simulink model "IMUdataFinalr3PDs0x2810x29"  (R2024a)
settings: Solver=FixedStepAuto  StartTime=0.0  StopTime=100  FixedStep=.01  RelTol=1e-3  EnableMultiTasking=on
libraries: instrumentlib x2, hdlsllib x1, instrumentseriallib x1
settings Model: Creator=juanandrespelaezb  LastModifiedBy=NYCST
settings SolverCC: PositivePriorityOrder=on  AutoInsertRateTranBlk=on
settings OptimizationCC: EnhancedBackFolding=on  PassReuseOutputArgsThreshold=0  MaxStackSize=64  OptimizeBlockOrder=speed  DifferentSizesBufferReuse=on  OptimizationCustomize=off
settings DebuggingCC: ParameterTunabilityLossMsg=error
settings HardwareCC: ProdBitPerLong=64  ProdLargestAtomicInteger=LongLong  ProdLargestAtomicFloat=Double  ProdLongLongMode=on  ProdHWDeviceType=ARM Compatible->ARM 64-bit (LP64)
settings RTWCC: Description=Embedded Coder  SystemTargetFile=ert.tlc  HardwareBoard=Raspberry Pi (64bit)  TLCOptions="-aInlineSetEventsForThisBaseRateFcn=TLC_FALSE -aSuppressMultiTaskScheduler=TLC_FALSE  -aRateBasedStepFcn=0"  TemplateMakefile=ert_default_tmf  Toolchain=GNU GCC Embedded Linux  BuildConfiguration=Faster Runs
settings CodeAppCC: ForceParamTrailComments=on  OperatorAnnotations=on
settings ERTTargetCC: ERTCustomFileBanners=off  SupportContinuousTime=on  SupportNonInlinedSFcns=on  RemoveResetFunc=off  SupportVariableSizeSignals=on  ModelStepFunctionPrototypeControlCompliant=off  ExtModeTransport=2  ExtModeStaticAlloc=on  ExtModeMexFile=ext_xcp  ExtModeIntrfLevel=Level2 - Open

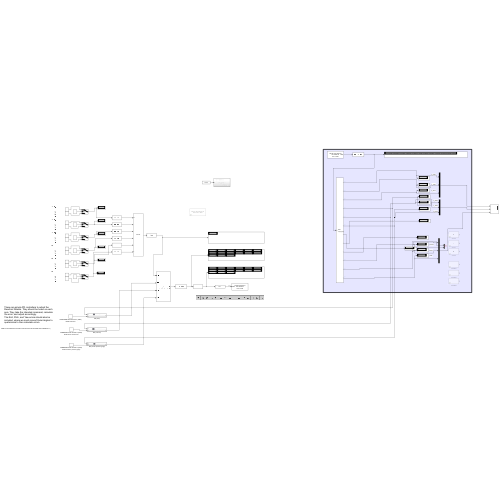
[thumbnail: Simulink's stored preview of the top-level diagram]
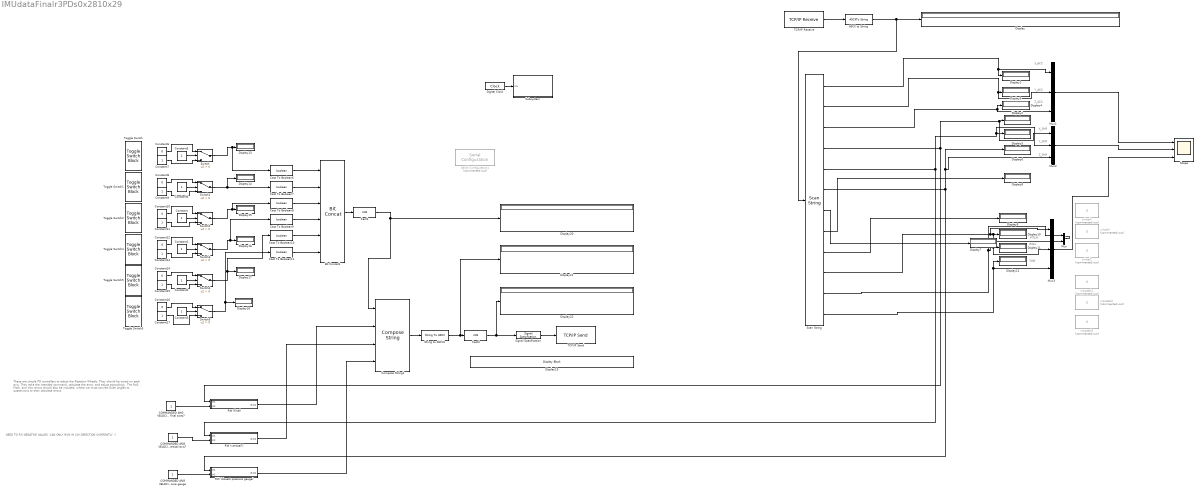
== system IMUdataFinalr3PDs0x2810x29 ==
  note: NEED TO FIX NEGATIVE VALUES. CAN ONLY RUN IN CW DIRECTION CURRENTLY :(
  note: These are simple PD controllers to adjust the Reaction Wheels. They should be tuned on each axis. They take the intended command, calculate the error, and adjust accordingly.
      | The Roll, Pitch, and Yaw errors should also be included, where we must convert Euler Angles to quaternions to then calculate errors.
  note: ROLL
  note: Z_GYR
  note: PITCH
  note: YAW
  note: Y_GYR
  note: X_GYR
  note: Z_ACC
  note: Y_ACC
  note: X_ACC
  ASCII to String : ASCIIToString
  Bit Concat1 : hdlsllib/Logic and Bit Operations/Bit Concat  numInputs=6
  COMMANDED ANG VELOCITY (PWM) IN RW about vertical axis? : Constant
  COMMANDED ANG VELOCITY (PWM) IN RW closest to pressure gauge : Constant
  COMMANDED ANG VELOCITY (PWM) IN RW final axes? : Constant
  Cast To Boolean{6..11} (6 alike) : DataTypeConversion  OutDataTypeStr=boolean  SaturateOnIntegerOverflow=off  RndMeth=Floor
  Cast1 : DataTypeConversion  OutDataTypeStr=int8  SaturateOnIntegerOverflow=off  RndMeth=Floor
  Cast4 : DataTypeConversion  OutDataTypeStr=int8  SaturateOnIntegerOverflow=off  RndMeth=Floor
  Compose String1 : ComposeString  Format="\"%02d;%03d;%03d;%03d\\n\""
  Constant{,1..5,7,9,11,13,15,17} (12 alike) : Constant
  Constant{6,8,10,12,14,16} (6 alike) : Constant  Value=0
  Digital Clock : DigitalClock
  Display{,1..18,20..22} (22 alike) : Display
  Display19 : DisplayBlock  LabelPosition=Hide  Format=long  Transparency=1
  Mux : Mux  Inputs=2
  Mux1 : Mux  Inputs=3
  Mux2 : Mux  Inputs=3
  Mux3 : Mux  Inputs=3
  RW (closest pressure gauge) : Subsystem
  RW (final) : Subsystem
  RW (vertical?) : Subsystem
  Scan String : ScanString  Format="\"%f,%f,%f,%f,%f,%f,%f,%f,%f,%f,%f,%f\""
  Scope : Scope  NumInputPorts=3
  Serial Configuration1 : instrumentseriallib/Serial Configuration  Priority=-200000  Commented=on  PortSel=/dev/cu.usbmodem2101  Port=/dev/cu.usbmodem2101  ComPort=/dev/cu.usbmodem2101  BaudRate=9600  DataBits=8  Parity=none  StopBits=1  ByteOrder=little-endian  FlowControl=none  Timeout=10  SimulateUsing=Interpreted execution  BlockInModel=on  aMode=1
  Signal Specification : SignalSpecification  SampleTime=.1
      settings: LockScale=on
  String to ASCII1 : StringToASCII  OutputVectorSize=15
  Subsystem : Subsystem
  Switch{,1..5} (6 alike) : Switch  Criteria=u2 > Threshold  SaturateOnIntegerOverflow=off  InputSameDT=off
  TCP/IP Receive : instrumentlib/TCP//IP Receive  Host=192.168.86.21  Port=12345  DataSize=[ 120, 1 ]  DataType=uint8  ASCIIFormatting=%f  Terminator=LF  CustomTerminator=10  ByteOrder=big-endian  EnableBlockingMode=on  Timeout=10  SampleTime=0.01  SimulateUsing=Interpreted execution
  TCP/IP Send : instrumentlib/TCP//IP Send  Host=192.168.86.21  Port=12345  ByteOrder=big-endian  EnableBlockingMode=on  Timeout=10  TransferDelay=on  SimulateUsing=Interpreted execution
  Toggle Switch{,1..5} (6 alike) : ToggleSwitchBlock
      settings: Values={{'Off', 'On'}, [0 1]}
  massBal1 : Constant  Commented=on  Value=0
  massBal2 : Constant  Commented=on  Value=0
  massBal3 : Constant  Commented=on  Value=0
  wheelX : Constant  Commented=on  Value=0
  wheelY : Constant  Commented=on  Value=0
  wheelZ : Constant  Commented=on  Value=0
  wires:
  Mux/1 -> ?
  Scan String/2 -> Mux1/2, Display3/1
  ASCII to String/1 -> Scan String/1, Display/1
  Scan String/7 -> Display7/1
  Scan String/1 -> Display1/1, Mux1/1
  Mux2/1 -> Scope/2
  Scan String/11 -> Mux/1, Mux3/2, Display11/1
  Mux1/1 -> Scope/1
  Scan String/6 -> Mux2/3, Display6/1, RW (closest pressure gauge)/1(In1)
  Scan String/3 -> Mux1/3, Display4/1
  Scan String/5 -> RW (vertical?)/1(In1), Mux2/2, Display5/1
  Scan String/8 -> Display8/1
  Scan String/4 -> RW (final)/1(In1), Display2/1, Mux2/1
  Scan String/9 -> Display9/1
  Scan String/12 -> Display12/1, Mux3/3
  Scan String/10 -> Mux3/1, Mux/2, Display10/1
  Digital Clock/1 -> Subsystem/1(In1)
  TCP/IP Receive/1 -> ASCII to String/1
  Constant6/1 -> Switch/1
  Constant7/1 -> Switch/3
  Constant8/1 -> Switch1/1
  Constant9/1 -> Switch1/3
  Constant10/1 -> Switch2/1
  Constant11/1 -> Switch2/3
  Constant13/1 -> Switch3/3
  Constant12/1 -> Switch3/1
  Constant14/1 -> Switch4/1
  Constant15/1 -> Switch4/3
  Constant16/1 -> Switch5/1
  Constant17/1 -> Switch5/3
  Constant/1 -> Switch2/2
  Constant1/1 -> Switch3/2
  Constant2/1 -> Switch4/2
  Constant3/1 -> Switch5/2
  Constant4/1 -> Switch1/2
  Constant5/1 -> Switch/2
  Switch/1 -> Cast To Boolean6/1, Display13/1
  Switch1/1 -> Cast To Boolean7/1, Display14/1
  Switch2/1 -> Cast To Boolean8/1, Display15/1
  Switch3/1 -> Cast To Boolean9/1, Display16/1
  Switch4/1 -> Cast To Boolean10/1, Display17/1
  Switch5/1 -> Cast To Boolean11/1, Display18/1
  Cast To Boolean9/1 -> Bit Concat1/4
  Cast To Boolean7/1 -> Bit Concat1/2
  Cast To Boolean10/1 -> Bit Concat1/5
  Cast To Boolean6/1 -> Bit Concat1/1
  Cast To Boolean8/1 -> Bit Concat1/3
  Cast To Boolean11/1 -> Bit Concat1/6
  Bit Concat1/1 -> Cast1/1
  Cast1/1 -> Compose String1/1, Display20/1
  Compose String1/1 -> String to ASCII1/1
  String to ASCII1/1 -> Display21/1, Cast4/1
  Cast4/1 -> Display22/1, Signal Specification/1
  Signal Specification/1 -> TCP/IP Send/1
  Mux3/1 -> Scope/3
  COMMANDED ANG VELOCITY (PWM) IN RW closest to pressure gauge/1 -> RW (closest pressure gauge)/2(In2)
  RW (closest pressure gauge)/1(Out1) -> Compose String1/4
  COMMANDED ANG VELOCITY (PWM) IN RW about vertical axis?/1 -> RW (vertical?)/2(In2)
  RW (vertical?)/1(Out1) -> Compose String1/3
  COMMANDED ANG VELOCITY (PWM) IN RW final axes?/1 -> RW (final)/2(In2)
  RW (final)/1(Out1) -> Compose String1/2

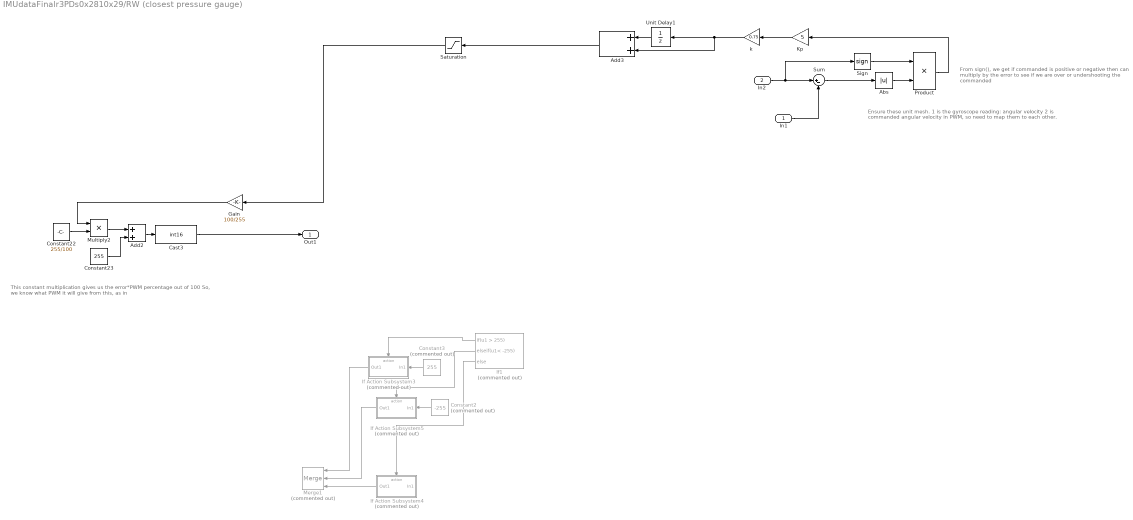
== system IMUdataFinalr3PDs0x2810x29/RW (closest pressure gauge) ==
  note: This constant multiplication gives us the error*PWM percentage out of 100
      | So, we know what PWM it will give from this, as in
  note: From sign(), we get if commanded is positive or negative
      | then can multiply by the error to see if we are over or undershooting
      | the commanded
  note: Ensure these unit mesh. 1 is the gyroscope reading: angular velocity
      | 2 is commanded angular velocity in PWM, so need to map them to each other.
  In1 : Inport
  In2 : Inport  Port=2
  Abs : Abs  SaturateOnIntegerOverflow=off
  Add2 : Sum
  Add3 : Sum
  Cast3 : DataTypeConversion  OutDataTypeStr=int16  SaturateOnIntegerOverflow=off  RndMeth=Floor
  Constant2 : Constant  Commented=on  Value=-255
  Constant22 : Constant  Value=255/100
  Constant23 : Constant  Value=255
  Constant3 : Constant  Commented=on  Value=255
  Gain : Gain  Gain=100/255
  If Action Subsystem3 : Subsystem  Commented=on  TreatAsAtomicUnit=on
  If Action Subsystem4 : Subsystem  Commented=on  TreatAsAtomicUnit=on
  If Action Subsystem5 : Subsystem  Commented=on  TreatAsAtomicUnit=on
  If1 : If  Commented=on  IfExpression=u1 > 255  ElseIfExpressions=u1< -255
  Kp : Gain  Gain=5
  Merge1 : Merge  Commented=on  Inputs=3
  Multiply2 : Product
  Product : Product
  Saturation : Saturate  UpperLimit=255  LowerLimit=-255
  Sign : Signum
  Sum : Sum  Inputs=|+-
  Unit Delay1 : UnitDelay  SampleTime=-1  HasFrameUpgradeWarning=on
  k : Gain  Gain=0.75
  Out1 : Outport
  wires:
  Multiply2/1 -> Add2/1
  Gain/1 -> Multiply2/1
  Constant23/1 -> Add2/2
  k/1 -> Add3/2, Unit Delay1/1
  Sum/1 -> Abs/1
  Unit Delay1/1 -> Add3/1
  Add2/1 -> Cast3/1
  Constant22/1 -> Multiply2/2
  Saturation/1 -> Gain/1
  Kp/1 -> k/1
  In1/1 -> Sum/2
  Cast3/1 -> Out1/1
  In2/1 -> Sign/1, Sum/1
  Sign/1 -> Product/1
  Abs/1 -> Product/2
  Product/1 -> Kp/1
  If1/2 -> If Action Subsystem5/Action
  Constant2/1 -> If Action Subsystem5/1(In1)
  Constant3/1 -> If Action Subsystem3/1(In1)
  If1/1 -> If Action Subsystem3/Action
  If Action Subsystem5/1(Out1) -> Merge1/2
  ? -> If Action Subsystem4/1(In1), If1/1
  If Action Subsystem3/1(Out1) -> Merge1/1
  If1/3 -> If Action Subsystem4/Action
  If Action Subsystem4/1(Out1) -> Merge1/3
  Add3/1 -> Saturation/1

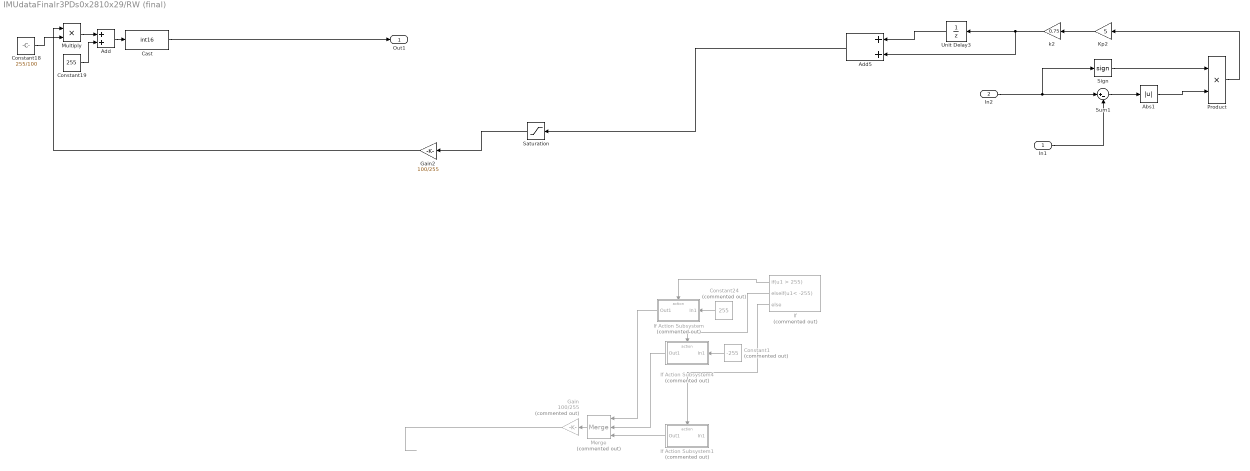
== system IMUdataFinalr3PDs0x2810x29/RW (final) ==
  In1 : Inport
  In2 : Inport  Port=2
  Abs1 : Abs  SaturateOnIntegerOverflow=off
  Add : Sum
  Add5 : Sum
  Cast : DataTypeConversion  OutDataTypeStr=int16  SaturateOnIntegerOverflow=off  RndMeth=Floor
  Constant1 : Constant  Commented=on  Value=-255
  Constant18 : Constant  Value=255/100
  Constant19 : Constant  Value=255
  Constant24 : Constant  Commented=on  Value=255
  Gain : Gain  Commented=on  Gain=100/255
  Gain2 : Gain  Gain=100/255
  If : If  Commented=on  IfExpression=u1 > 255  ElseIfExpressions=u1< -255
  If Action Subsystem : Subsystem  Commented=on  TreatAsAtomicUnit=on
  If Action Subsystem1 : Subsystem  Commented=on  TreatAsAtomicUnit=on
  If Action Subsystem4 : Subsystem  Commented=on  TreatAsAtomicUnit=on
  Kp2 : Gain  Gain=5
  Merge : Merge  Commented=on  Inputs=3
  Multiply : Product
  Product : Product
  Saturation : Saturate  UpperLimit=255  LowerLimit=-255
  Sign : Signum
  Sum1 : Sum  Inputs=|+-
  Unit Delay3 : UnitDelay  SampleTime=-1  HasFrameUpgradeWarning=on
  k2 : Gain  Gain=0.75
  Out1 : Outport
  wires:
  Constant19/1 -> Add/2
  Constant18/1 -> Multiply/2
  Unit Delay3/1 -> Add5/1
  Multiply/1 -> Add/1
  Saturation/1 -> Gain2/1
  Add/1 -> Cast/1
  In2/1 -> Sign/1, Sum1/1
  Kp2/1 -> k2/1
  Cast/1 -> Out1/1
  k2/1 -> Add5/2, Unit Delay3/1
  Sum1/1 -> Abs1/1
  In1/1 -> Sum1/2
  Gain2/1 -> Multiply/1
  Gain/1 -> ?
  If/3 -> If Action Subsystem1/Action
  If Action Subsystem/1(Out1) -> Merge/1
  Merge/1 -> Gain/1
  If Action Subsystem4/1(Out1) -> Merge/2
  If/2 -> If Action Subsystem4/Action
  ? -> If Action Subsystem1/1(In1)
  If Action Subsystem1/1(Out1) -> Merge/3
  Constant1/1 -> If Action Subsystem4/1(In1)
  ? -> If/1
  Constant24/1 -> If Action Subsystem/1(In1)
  If/1 -> If Action Subsystem/Action
  Product/1 -> Kp2/1
  Sign/1 -> Product/1
  Abs1/1 -> Product/2
  Add5/1 -> Saturation/1

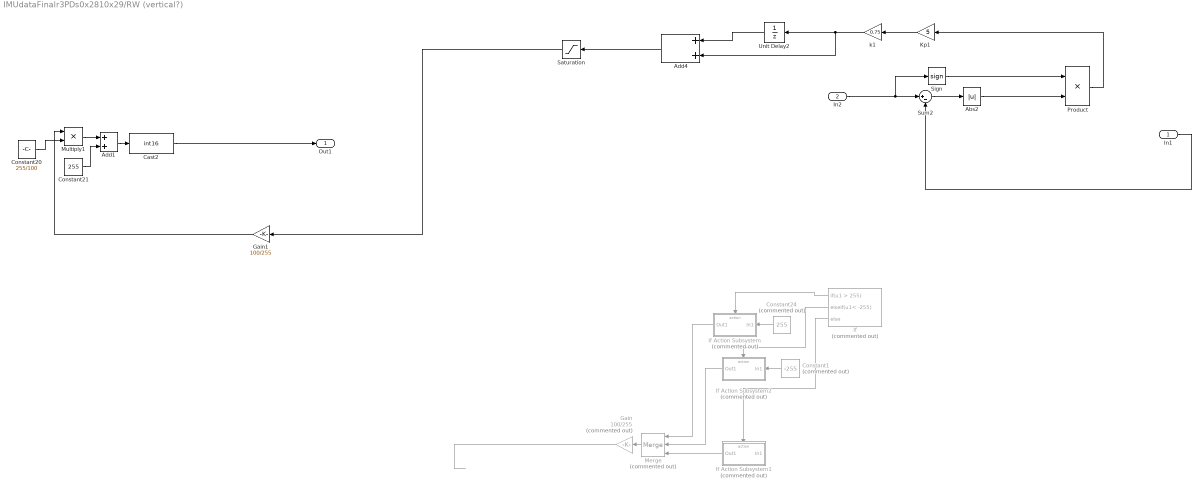
== system IMUdataFinalr3PDs0x2810x29/RW (vertical?) ==
  In1 : Inport
  In2 : Inport  Port=2
  Abs2 : Abs  SaturateOnIntegerOverflow=off
  Add1 : Sum
  Add4 : Sum
  Cast2 : DataTypeConversion  OutDataTypeStr=int16  SaturateOnIntegerOverflow=off  RndMeth=Floor
  Constant1 : Constant  Commented=on  Value=-255
  Constant20 : Constant  Value=255/100
  Constant21 : Constant  Value=255
  Constant24 : Constant  Commented=on  Value=255
  Gain : Gain  Commented=on  Gain=100/255
  Gain1 : Gain  Gain=100/255
  If : If  Commented=on  IfExpression=u1 > 255  ElseIfExpressions=u1< -255
  If Action Subsystem : Subsystem  Commented=on  TreatAsAtomicUnit=on
  If Action Subsystem1 : Subsystem  Commented=on  TreatAsAtomicUnit=on
  If Action Subsystem2 : Subsystem  Commented=on  TreatAsAtomicUnit=on
  Kp1 : Gain  Gain=5
  Merge : Merge  Commented=on  Inputs=3
  Multiply1 : Product
  Product : Product
  Saturation : Saturate  UpperLimit=255  LowerLimit=-255
  Sign : Signum
  Sum2 : Sum  Inputs=|+-
  Unit Delay2 : UnitDelay  SampleTime=-1  HasFrameUpgradeWarning=on
  k1 : Gain  Gain=0.75
  Out1 : Outport
  wires:
  Constant20/1 -> Multiply1/2
  Multiply1/1 -> Add1/1
  Constant21/1 -> Add1/2
  Gain1/1 -> Multiply1/1
  In2/1 -> Sign/1, Sum2/1
  k1/1 -> Add4/2, Unit Delay2/1
  Unit Delay2/1 -> Add4/1
  Sum2/1 -> Abs2/1
  Add1/1 -> Cast2/1
  Kp1/1 -> k1/1
  Saturation/1 -> Gain1/1
  Cast2/1 -> Out1/1
  In1/1 -> Sum2/2
  Product/1 -> Kp1/1
  Abs2/1 -> Product/2
  Sign/1 -> Product/1
  If/2 -> If Action Subsystem2/Action
  Constant1/1 -> If Action Subsystem2/1(In1)
  Constant24/1 -> If Action Subsystem/1(In1)
  If/1 -> If Action Subsystem/Action
  ? -> If Action Subsystem1/1(In1)
  If Action Subsystem2/1(Out1) -> Merge/2
  ? -> If/1
  Gain/1 -> ?
  If Action Subsystem/1(Out1) -> Merge/1
  Merge/1 -> Gain/1
  If/3 -> If Action Subsystem1/Action
  If Action Subsystem1/1(Out1) -> Merge/3
  Add4/1 -> Saturation/1

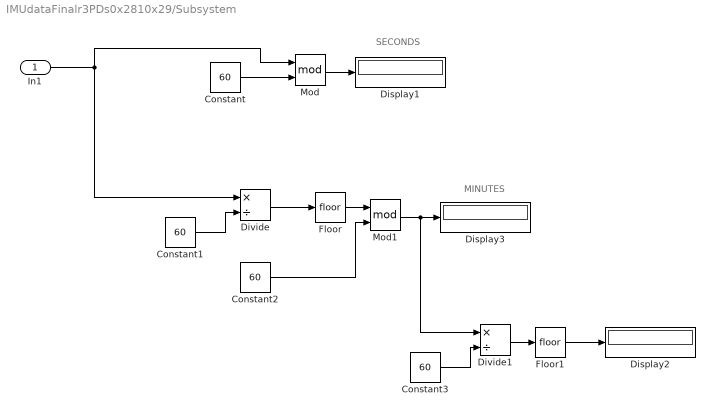
== system IMUdataFinalr3PDs0x2810x29/Subsystem ==
  note: SECONDS
  note: MINUTES
  In1 : Inport
  Constant{,1..3} (4 alike) : Constant  Value=60
  Display1 : Display
  Display2 : Display
  Display3 : Display
  Divide : Product  Inputs=*/
  Divide1 : Product  Inputs=*/
  Floor : Rounding
  Floor1 : Rounding
  Mod : Math  Operator=mod  SignedPower=on
  Mod1 : Math  Operator=mod  SignedPower=on
  wires:
  Constant/1 -> Mod/2
  Mod/1 -> Display1/1
  In1/1 -> Divide/1, Mod/1
  Constant1/1 -> Divide/2
  Divide/1 -> Floor/1
  Floor/1 -> Mod1/1
  Constant2/1 -> Mod1/2
  Mod1/1 -> Divide1/1, Display3/1
  Constant3/1 -> Divide1/2
  Divide1/1 -> Floor1/1
  Floor1/1 -> Display2/1

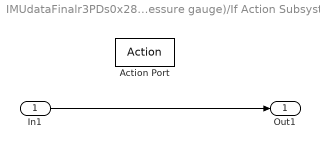
== system IMUdataFinalr3PDs0x2810x29/RW (closest pressure gauge)/If Action Subsystem3 ==
  In1 : Inport
  Action Port : ActionPort  ActionPortLabel=if(u1 > 255)
  Out1 : Outport
  wires:
  In1/1 -> Out1/1

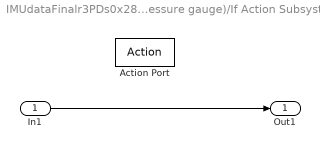
== system IMUdataFinalr3PDs0x2810x29/RW (closest pressure gauge)/If Action Subsystem4 ==
  In1 : Inport
  Action Port : ActionPort  ActionPortLabel=else
  Out1 : Outport
  wires:
  In1/1 -> Out1/1

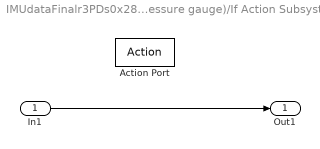
== system IMUdataFinalr3PDs0x2810x29/RW (closest pressure gauge)/If Action Subsystem5 ==
  In1 : Inport
  Action Port : ActionPort  ActionPortLabel=elseif(u1< -255)
  Out1 : Outport
  wires:
  In1/1 -> Out1/1

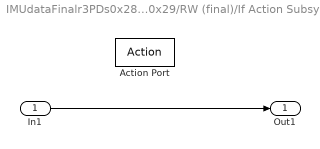
== system IMUdataFinalr3PDs0x2810x29/RW (final)/If Action Subsystem ==
  In1 : Inport
  Action Port : ActionPort  ActionPortLabel=if(u1 > 255)
  Out1 : Outport
  wires:
  In1/1 -> Out1/1

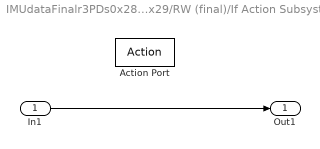
== system IMUdataFinalr3PDs0x2810x29/RW (final)/If Action Subsystem1 ==
  In1 : Inport
  Action Port : ActionPort  ActionPortLabel=else
  Out1 : Outport
  wires:
  In1/1 -> Out1/1

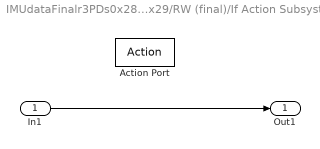
== system IMUdataFinalr3PDs0x2810x29/RW (final)/If Action Subsystem4 ==
  In1 : Inport
  Action Port : ActionPort  ActionPortLabel=elseif(u1< -255)
  Out1 : Outport
  wires:
  In1/1 -> Out1/1

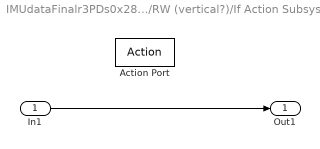
== system IMUdataFinalr3PDs0x2810x29/RW (vertical?)/If Action Subsystem ==
  In1 : Inport
  Action Port : ActionPort  ActionPortLabel=if(u1 > 255)
  Out1 : Outport
  wires:
  In1/1 -> Out1/1

== system IMUdataFinalr3PDs0x2810x29/RW (vertical?)/If Action Subsystem1 ==
  In1 : Inport
  Action Port : ActionPort  ActionPortLabel=else
  Out1 : Outport
  wires:
  In1/1 -> Out1/1

== system IMUdataFinalr3PDs0x2810x29/RW (vertical?)/If Action Subsystem2 ==
  In1 : Inport
  Action Port : ActionPort  ActionPortLabel=elseif(u1< -255)
  Out1 : Outport
  wires:
  In1/1 -> Out1/1
